simulink model "controller_velocity_LQR"  (R2021a)
settings: Solver=FixedStepAuto  StartTime=0.0  StopTime=10.0  RelTol=1e-3
undefined symbols (not defined in the file): DiscIntNeverNeededParam, g, hover_init, LQR, max_total_T, Ts_mpc
settings Model: Creator=esl  LastModifiedBy=esl

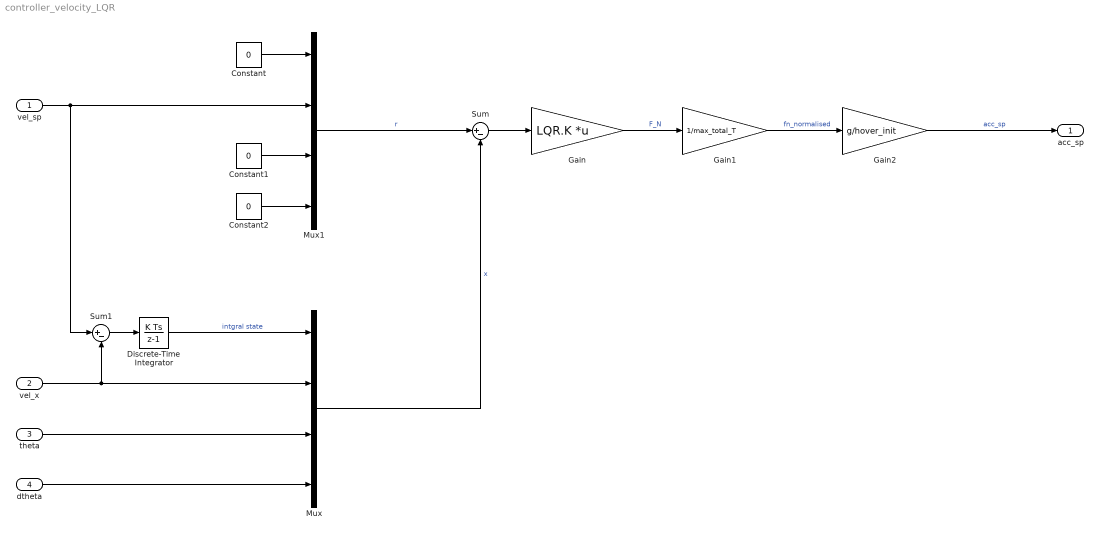
== system controller_velocity_LQR ==
  vel_sp : Inport  OutDataTypeStr=double  PortDimensions=num_axis
  vel_x : Inport  Port=2  OutDataTypeStr=double  PortDimensions=1
  theta : Inport  Port=3  OutDataTypeStr=double  PortDimensions=1
  dtheta : Inport  Port=4  OutDataTypeStr=double  PortDimensions=1
  Constant : Constant  Value=0
  Constant1 : Constant  Value=0
  Constant2 : Constant  Value=0
  Discrete-Time Integrator : DiscreteIntegrator  SampleTime=Ts_mpc  ICPrevOutput=DiscIntNeverNeededParam  ICPrevScaledInput=DiscIntNeverNeededParam
  Gain : Gain  Gain=LQR.K  Multiplication=Matrix(K*u) (u vector)
  Gain1 : Gain  Gain=1/max_total_T
  Gain2 : Gain  Gain=g/hover_init
  Mux : Mux
  Mux1 : Mux
  Sum : Sum  Inputs=|+-
  Sum1 : Sum  Inputs=|+-
  acc_sp : Outport  OutDataTypeStr=double  PortDimensions=1
  wires:
  Mux1/1 -> Sum/1  "r"
  Mux/1 -> Sum/2  "x"
  Sum/1 -> Gain/1
  Gain/1 -> Gain1/1  "F_N"
  Discrete-Time Integrator/1 -> Mux/1  "intgral state"
  vel_x/1 -> Sum1/2, Mux/2
  theta/1 -> Mux/3
  Constant2/1 -> Mux1/4
  Constant1/1 -> Mux1/3
  Constant/1 -> Mux1/1
  vel_sp/1 -> Sum1/1, Mux1/2
  Sum1/1 -> Discrete-Time Integrator/1
  Gain1/1 -> Gain2/1  "fn_normalised"
  Gain2/1 -> acc_sp/1  "acc_sp"
  dtheta/1 -> Mux/4
